simulink model "suspension_model"  (R2023b)
settings: Solver=VariableStepAuto  StartTime=0.0  StopTime=10.0  RelTol=1e-3
InitFcn:
  | suspension_params
values from neighbouring files (symbols this model uses):
  h_0 = 0    [suspension_params.m]
  h_bump = 0.03    [suspension_params.m]
  T = F_tot * r_wheel    [drive_train_analysis.m]    (also in suspension_params.m = 20; torsion_bar_analysis.m = F * r * cos(alpha))
  t_bump = w_bump/v    (= 0.06)    [suspension_params.m]
  t_delay = (l1 - l2)/v    (= 0.4)    [suspension_params.m]
  t_offset = 2    [suspension_params.m]
libraries: simulink x1
settings Model: Creator=micha  LastModifiedBy=micha

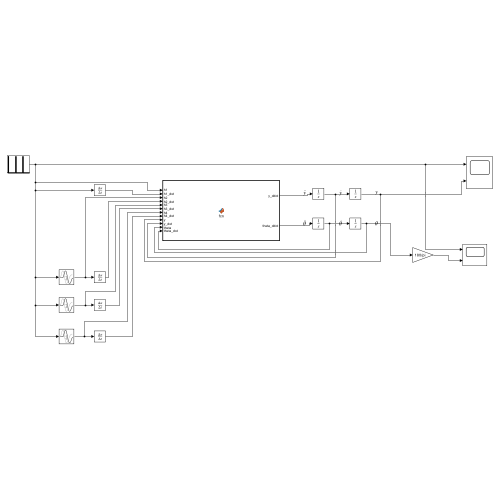
[thumbnail: Simulink's stored preview of the top-level diagram]
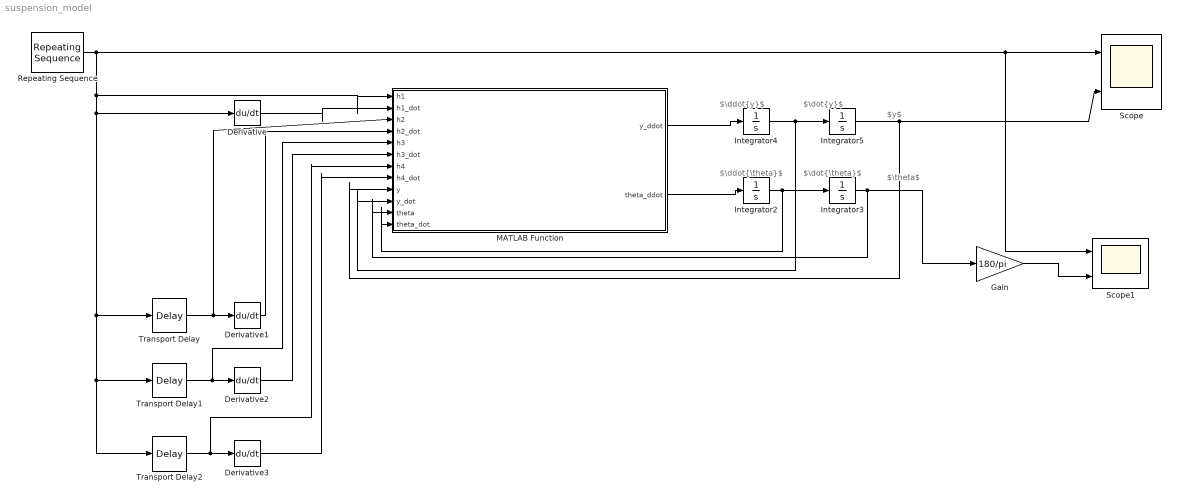
== system suspension_model ==
  note: $\ddot{\theta}$
  note: $\dot{\theta}$
  note: $\ddot{y}$
  note: $\dot{y}$
  note: $y$
  note: $\theta$
  Derivative{,1..3} (4 alike) : Derivative
  Gain : Gain  Gain=180/pi
  Integrator{2..5} (4 alike) : Integrator
  MATLAB Function : MATLAB Function  TreatAsAtomicUnit=on
  Repeating Sequence : simulink/Sources/Repeating Sequence  rep_seq_t="[0 t_offset t_offset+t_bump*0.2  t_offset+t_bump*0.8 t_offset+t_bump T]"  rep_seq_y=[h_0 h_0 h_bump h_bump h_0 0]
  Scope : Scope  NumInputPorts=2
  Scope1 : Scope  NumInputPorts=2
  Transport Delay : TransportDelay  DelayTime=t_delay
  Transport Delay1 : TransportDelay  DelayTime=2*t_delay
  Transport Delay2 : TransportDelay  DelayTime=3*t_delay
  wires:
  Repeating Sequence/1 -> Transport Delay2/1, Transport Delay1/1, Transport Delay/1, Derivative/1, MATLAB Function/1(h1), Scope1/1, Scope/1
  Integrator2/1 -> Integrator3/1, MATLAB Function/12(theta_dot)
  MATLAB Function/2(theta_ddot) -> Integrator2/1
  MATLAB Function/1(y_ddot) -> Integrator4/1
  Integrator4/1 -> MATLAB Function/10(y_dot), Integrator5/1
  Integrator5/1 -> Scope/2, MATLAB Function/9(y)
  Derivative/1 -> MATLAB Function/2(h1_dot)
  Transport Delay/1 -> Derivative1/1, MATLAB Function/3(h2)
  Derivative1/1 -> MATLAB Function/4(h2_dot)
  Integrator3/1 -> Gain/1, MATLAB Function/11(theta)
  Gain/1 -> Scope1/2
  Transport Delay1/1 -> MATLAB Function/5(h3), Derivative2/1
  Derivative2/1 -> MATLAB Function/6(h3_dot)
  Transport Delay2/1 -> MATLAB Function/7(h4), Derivative3/1
  Derivative3/1 -> MATLAB Function/8(h4_dot)

== matlab function suspension_model/MATLAB Function ==
  data: h1 input; y_ddot output; theta_ddot output; h1_dot input; h2 input; h2_dot input; h3 input; h3_dot input; h4 input; h4_dot input; y input; y_dot input; theta input; theta_dot input
function [y_ddot, theta_ddot] = fcn(h1, h1_dot, h2, h2_dot, h3, h3_dot, h4, h4_dot, y, y_dot, theta, theta_dot)

g = 9.8;
m = 100;
Hv = 0.2; % height of vehicle
L = 0.8; % length of vehicle
l1 = L * (3/8); % wheel placement
l2 = L * (1/8);
l3 = -l2;
l4 = -l1;
I = 1/12 * m * (Hv^2 + L^2);

H = [h1, h2, h3, h4]; % vertical wheel heigts
H_dot = [h1_dot, h2_dot, h3_dot, h4_dot]; % vertical wheel velocities
k_sus = 8000;
c_sus = k_sus/2;
K = [k_sus, k_sus, k_sus, k_sus]; % wheel suspension spring constants
C = [c_sus, c_sus, c_sus, c_sus]; % wheel suspension damping constants
l = [l1, l2, l3, l4]; % wheel placement distances

y_ddot = 0;
theta_ddot = 0;

for i = 1:length(H)
    F = K(i) * (H(i) - (y + l(i) * theta)) + C(i) * (H_dot(i) - (y_dot + l(i) * theta_dot));
    
    y_ddot = y_ddot + F/m;
    theta_ddot = theta_ddot + (F * l(i))/I;
end
